simulink model "energy_detect_th"  (R2022b)
settings: Solver=VariableStepAuto  StartTime=0.0  StopTime=2  RelTol=1e-3
settings Model: Creator=Lenovo  LastModifiedBy=Lenovo

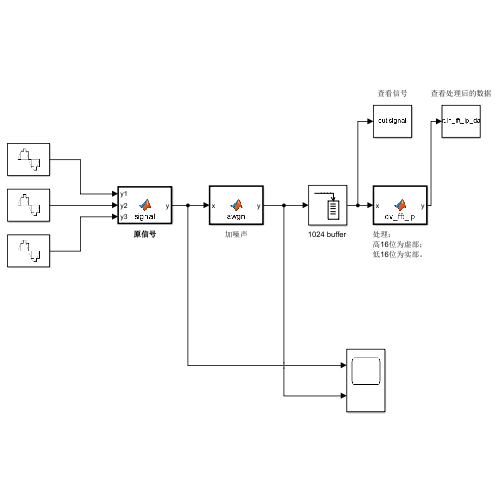
[thumbnail: Simulink's stored preview of the top-level diagram]
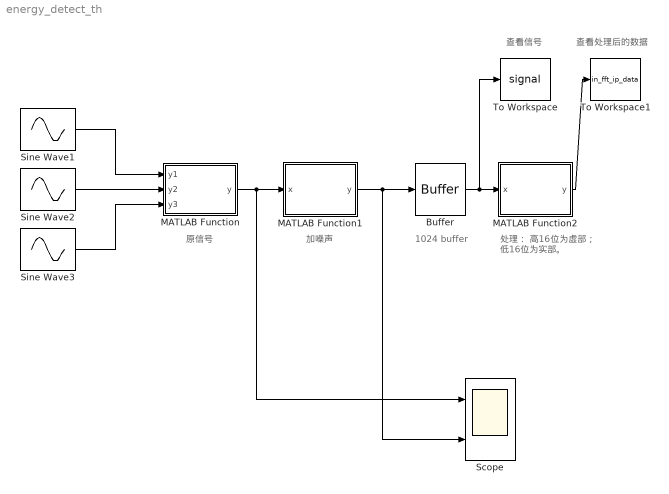
== system energy_detect_th ==
  note: 原信号
  note: 加噪声
  note: 1024 buffer
  note: 处理：
      | 高16位为虚部；
      | 低16位为实部。
  note: 查看信号
  note: 查看处理后的数据
  Buffer : Buffer  N=1024  OutputFrames=off
  MATLAB Function : MATLAB Function  TreatAsAtomicUnit=on
  MATLAB Function1 : MATLAB Function  TreatAsAtomicUnit=on
  MATLAB Function2 : MATLAB Function  TreatAsAtomicUnit=on
  Scope : Scope  NumInputPorts=2
  Sine Wave1 : Sin  Amplitude=10  Frequency=628  SampleTime=0.001
  Sine Wave2 : Sin  Amplitude=10  Frequency=1257  SampleTime=0.001
  Sine Wave3 : Sin  Amplitude=10  Frequency=1885  SampleTime=0.001
  To Workspace : ToWorkspace  VariableName=signal  SampleTime=-1
      settings: Save2DSignal=2-D array (concatenate along first dimension)
  To Workspace1 : ToWorkspace  VariableName=in_fft_ip_data  SampleTime=-1
      settings: Save2DSignal=2-D array (concatenate along first dimension)
  wires:
  Sine Wave1/1 -> MATLAB Function/1(y1)
  Sine Wave2/1 -> MATLAB Function/2(y2)
  Sine Wave3/1 -> MATLAB Function/3(y3)
  MATLAB Function/1(y) -> Scope/1, MATLAB Function1/1(x)
  MATLAB Function1/1(y) -> Buffer/1, Scope/2
  Buffer/1 -> To Workspace/1, MATLAB Function2/1(x)
  MATLAB Function2/1(y) -> To Workspace1/1

== matlab function energy_detect_th/MATLAB Function ==
  data: y1 input; y output; y2 input; y3 input
function y = signal(y1, y2, y3)

y = y1 +  y2 + y3;

== matlab function energy_detect_th/MATLAB Function2 ==
  data: x input; y output
function y = dv_fft_ip(x)

real_x = int32(real(x));
imag_x = int32(imag(x));

y = int32(bitshift(imag_x, 16) + real_x);

== matlab function energy_detect_th/MATLAB Function1 ==
  data: x input; y output
function y = awgn(x)

y = awgn(x, 10, 'measured');
